simulink model "iq"  (R2021a)
settings: Solver=VariableStepAuto  StartTime=0.0  StopTime=0.2  FixedStep=1/150000  MaxStep=1e-6
undefined symbols (not defined in the file): in, ou
libraries: neural x55, spsMosfetLib x12, simulink x5, pid_lib x3, spsFirstOrderFilterLib x2, spsPermanentMagnetSynchronousMachineLib x2, spsCurrentMeasurementLib x2, spsDCVoltageSourceLib x2, spsThreePhaseVIMeasurementLib x2, spsabctoAlphaBetaZeroLib x2, spsabctodq0Lib x2, spsSVPWMGenerator2LevelLib x1
(part 1 of 5)
settings Model: Creator=Hassan Alam  LastModifiedBy=Omkar
settings SolverCC: ZeroCrossAlgorithm=Adaptive
settings DebuggingCC: MaskedZcDiagnostic=none  IgnoredZcDiagnostic=none  SFMachineParentedDataDiag=warning  ArithmeticOperatorsInVariantConditions=warning
settings SFSimCC: CustomCodeUndefinedFunction=UseInterfaceOnly

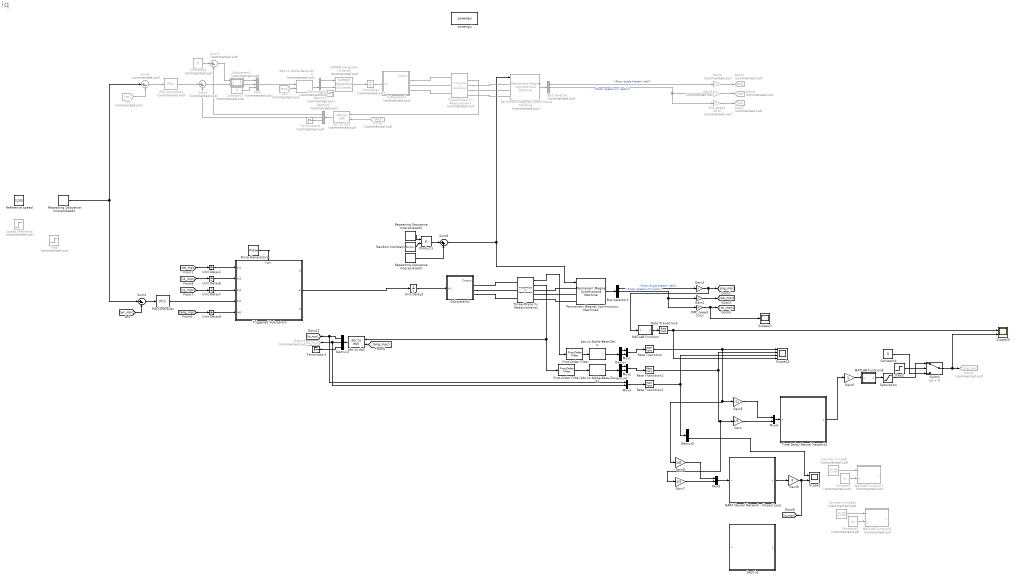
== system iq ==
  Bus Selector : BusSelector  Commented=on  OutputSignals=Rotor angle thetam (rad),Rotor speed wm (rad/s),Electromagnetic torque Te (N*m)
  Bus Selector1 : BusSelector  OutputSignals=Rotor angle thetam (rad),Rotor speed wm (rad/s),Electromagnetic torque Te (N*m)
  Constant : Constant  Commented=on  Value=in
  Constant1 : Constant  Commented=on  Value=0
  Constant2 : Constant  Commented=on  Value=0
  Constant3 : Constant  Commented=on  Value=ou
  Constant4 : Constant  Value=0
  Counter Limited : simulink/Sources/Counter Limited  Commented=on  uplimit=20000  tsamp=100e-6
  Counter Limited1 : simulink/Sources/Counter Limited  Commented=on  uplimit=20000  tsamp=10e-6
  Demux : Demux  Outputs=3
  Demux1 : Demux  Commented=on  Outputs=3
  Demux2 : Demux  Commented=on  Outputs=3
  Demux3 : Demux  Outputs=3
  Demux4 : Demux  Outputs=3
  Demux5 : Demux  Outputs=2
  FOC speed : Gain  Commented=on  Gain=30/pi
  First-Order Filter : spsFirstOrderFilterLib/First-Order Filter  FilterType=Lowpass  Tc=10e-5  Ts=0  Initialize=off  Vac_Init=[0, 0, 60]  Vdc_Init=0  PlotResponse=off  FreqRange="[0,  200,  1]"
  First-Order Filter1 : spsFirstOrderFilterLib/First-Order Filter  FilterType=Lowpass  Tc=10e-5  Ts=0  Initialize=off  Vac_Init=[0, 0, 60]  Vdc_Init=0  PlotResponse=off  FreqRange="[0,  200,  1]"
  From2 : From  Commented=on  GotoTag=ang
  Gain : Gain  Gain=1/3
  Gain1 : Gain  Commented=on  Gain=4
  Gain2 : Gain  Gain=4
  Gain3 : Gain  Gain=4
  Gain4 : Gain  Commented=on  Gain=4
  Gain5 : Gain  Gain=1/12
  Gain6 : Gain
  Gain7 : Gain  Gain=1/3
  Gain8 : Gain  Gain=1/8
  Gain9 : Gain  Gain=3
  Goto13 : Goto  Commented=on  GotoTag=iq_mpc
  Goto2 : Goto  Commented=on  GotoTag=ang
  Goto4 : Goto  Commented=on  GotoTag=we
  Goto6 : Goto  Commented=on  GotoTag=ang_mpc
  Goto7 : Goto  Commented=on  GotoTag=wr
  MATLAB Function : MATLAB Function  TreatAsAtomicUnit=on
  MATLAB Function1 : MATLAB Function  Commented=on  TreatAsAtomicUnit=on
  MATLAB Function2 : MATLAB Function  Commented=on  TreatAsAtomicUnit=on
  MATLAB Function5 : MATLAB Function  TreatAsAtomicUnit=on
  MPC speed : Gain  Gain=30/pi
  Mux : Mux  Commented=on  Inputs=3
  Mux{1..5} (5 alike) : Mux  Inputs=2
  NARX Neural Network - Closed Loop : Subsystem  mask{pi_input_1_delayed_1=[0;0;0;0], pi_input_1_delayed_2=[0;0;0;0], pi_input_1_delayed_3=[0;0;0;0], pi_input_1_delayed_4=[0;0;0;0], pi_input_1_delayed_5=[0;0;0;0], pi_input_1_delayed_6=[0;0;0;0], pi_input_1_delayed_7=[0;0;0;0], pi_input_1_delayed_8=[0;0;0;0], pi_input_1_delayed_9=[0;0;0;0], pi_input_1_delayed_10=[0;0;0;0], ai_layer_2_delayed_1=0, ai_layer_2_delayed_2=0, ai_layer_2_delayed_3=0, ai_layer_2_delayed_4=0, ai_layer_2_delayed_5=0, ai_layer_2_delayed_6=0, ai_layer_2_delayed_7=0, ai_layer_2_delayed_8=0, ai_layer_2_delayed_9=0, ai_layer_2_delayed_10=0}
      mask prompts: pi_input_1_delayed_1 "Preprocessed initial input 1 state at timestep 0."; pi_input_1_delayed_2 "Preprocessed initial input 1 state at timestep -1."; pi_input_1_delayed_3 "Preprocessed initial input 1 state at timestep -2."; pi_input_1_delayed_4 "Preprocessed initial input 1 state at timestep -3."; pi_input_1_delayed_5 "Preprocessed initial input 1 state at timestep -4."; pi_input_1_delayed_6 "Preprocessed initial input 1 state at timestep -5."; pi_input_1_delayed_7 "Preprocessed initial input 1 state at timestep -6."; pi_input_1_delayed_8 "Preprocessed initial input 1 state at timestep -7."; pi_input_1_delayed_9 "Preprocessed initial input 1 state at timestep -8."; pi_input_1_delayed_10 "Preprocessed initial input 1 state at timestep -9."; ai_layer_2_delayed_1 "Initial layer 2 state at timestep 0."; ai_layer_2_delayed_2 "Initial layer 2 state at timestep -1."; ai_layer_2_delayed_3 "Initial layer 2 state at timestep -2."; ai_layer_2_delayed_4 "Initial layer 2 state at timestep -3."; ai_layer_2_delayed_5 "Initial layer 2 state at timestep -4."; ai_layer_2_delayed_6 "Initial layer 2 state at timestep -5."; ai_layer_2_delayed_7 "Initial layer 2 state at timestep -6."; ai_layer_2_delayed_8 "Initial layer 2 state at timestep -7."; ai_layer_2_delayed_9 "Initial layer 2 state at timestep -8."; ai_layer_2_delayed_10 "Initial layer 2 state at timestep -9."
      mask help: NARX Neural Network - Closed Loop
      mask Display: e = 0.06;c1 = [120 150 230]/255;c2 = ([120 150 230]+0)/383;c3 = ([120 150 230]+128)/383;patch([0 1 1 0],[0 0 1 1],c1);patch([0 1 1 1-e 1-e 0+e],[0 0 1 1-e 0+e 0+e],c2);patch([0 0 1 1-e 0+e 0+e],[0 1 1 1-e 1-e 0+e],c3);plot([0 1 1 0 0],[0 0 1 1 0]);fprintf('NNET');port_label('input',1,' x');port_label('output',1,'y ');
  PID Controller : pid_lib/PID Controller  Controller=PI  Form=Parallel  TimeDomain=Discrete-time  UseExternalTs=off  SampleTime=1/2000  IntegratorMethod=Forward Euler  FilterMethod=Forward Euler  ControllerParametersSource=internal  P=0.02  I=20  D=0  UseFilter=on  N=100  TunerSelectOption=Transfer Function Based (PID Tuner App)  InitialConditionSource=internal  InitialConditionForIntegrator=0  InitialConditionForFilter=0  DifferentiatorICPrevScaledInput=0  ExternalReset=none  TrackingMode=off  Kt=1  LimitOutput=on  SatLimitsSource=internal  UpperSaturationLimit=3  LowerSaturationLimit=-3  LinearizeAsGain=on  AntiWindupMode=clamping  Kb=1  POutMin=[]  POutMax=[]  IOutMin=[]  IOutMax=[]  DOutMin=[]  DOutMax=[]  NOutMin=[]  NOutMax=[]  SumOutMin=[]  SumOutMax=[]  SaturationOutMin=[]  SaturationOutMax=[]  PParamMin=[]  PParamMax=[]  IParamMin=[]  IParamMax=[]  DParamMin=[]  DParamMax=[]  NParamMin=[]  NParamMax=[]  KbParamMin=[]  KbParamMax=[]  KtParamMin=[]  KtParamMax=[]  KbOutMin=[]  KbOutMax=[]  KtOutMin=[]  KtOutMax=[]  IntegratorOutMin=[]  IntegratorOutMax=[]  FilterOutMin=[]  FilterOutMax=[]  SumI1OutMin=[]  SumI1OutMax=[]  SumI2OutMin=[]  SumI2OutMax=[]  SumI3OutMin=[]  SumI3OutMax=[]  SumI4OutMin=[]  SumI4OutMax=[]  SumDOutMin=[]  SumDOutMax=[]  DifferentiatorOutMin=[]  DifferentiatorOutMax=[]  FilterDiffOutCoefMin=[]  FilterDiffOutCoefMax=[]  ReciprocalOutMin=[]  ReciprocalOutMax=[]  SumDenOutMin=[]  SumDenOutMax=[]  SumNumOutMin=[]  SumNumOutMax=[]  DivideOutMin=[]  DivideOutMax=[]  UdiffTsProdOutMin=[]  UdiffTsProdOutMax=[]  NTsProdOutMin=[]  NTsProdOutMax=[]  UintegralTsProdOutMin=[]  UintegralTsProdOutMax=[]  UngainTsProdOutMin=[]  UngainTsProdOutMax=[]  IntegratorContinuousStateAttributes=''  IntegratorStateMustResolveToSignalObject=off  IntegratorRTWStateStorageClass=Auto  FilterContinuousStateAttributes=''  FilterStateMustResolveToSignalObject=off  FilterRTWStateStorageClass=Auto  ParallelPVariant=InternalParameters  IdealPVariant=Disabled  IVariant=InternalParameters  DVariant=Disabled  IntegratorVariant=Discrete  SatVariant=Enabled  AWVariant=DiscClampingParallel  PCopyVariant=Disabled  TRVariant=Disabled  FdbkBlocksVariant=Forward  IdealPFdbkVariant=Disabled  SatFdbkVariant=Disabled  DerivativeFilterVariant=Disabled  NVariant=Disabled  NCopyVariant=Disabled_SignalSpec  FilterICVariant=Disabled  IntegratorICVariant=InternalICs  ExternalResetVariant=Disabled  TRSumVariant=Passthrough  SumFdbkVariant=Disabled  SumVariant=Sum_PI  TsampFilterVariant=InternalTs  TsampNgainVariant=Passthrough  TsampIntegralVariant=Passthrough  ExternalSaturationOutDataTypeStr=Inherit: Same as second input
  PID Controller1 : pid_lib/PID Controller  Commented=on  Controller=PI  Form=Parallel  TimeDomain=Discrete-time  UseExternalTs=off  SampleTime=1/2000  IntegratorMethod=Forward Euler  FilterMethod=Forward Euler  ControllerParametersSource=internal  P=0.02  I=20  D=0  UseFilter=on  N=100  TunerSelectOption=Transfer Function Based (PID Tuner App)  InitialConditionSource=internal  InitialConditionForIntegrator=0  InitialConditionForFilter=0  DifferentiatorICPrevScaledInput=0  ExternalReset=none  TrackingMode=off  Kt=1  LimitOutput=on  SatLimitsSource=internal  UpperSaturationLimit=3  LowerSaturationLimit=-3  LinearizeAsGain=on  AntiWindupMode=clamping  Kb=1  POutMin=[]  POutMax=[]  IOutMin=[]  IOutMax=[]  DOutMin=[]  DOutMax=[]  NOutMin=[]  NOutMax=[]  SumOutMin=[]  SumOutMax=[]  SaturationOutMin=[]  SaturationOutMax=[]  PParamMin=[]  PParamMax=[]  IParamMin=[]  IParamMax=[]  DParamMin=[]  DParamMax=[]  NParamMin=[]  NParamMax=[]  KbParamMin=[]  KbParamMax=[]  KtParamMin=[]  KtParamMax=[]  KbOutMin=[]  KbOutMax=[]  KtOutMin=[]  KtOutMax=[]  IntegratorOutMin=[]  IntegratorOutMax=[]  FilterOutMin=[]  FilterOutMax=[]  SumI1OutMin=[]  SumI1OutMax=[]  SumI2OutMin=[]  SumI2OutMax=[]  SumI3OutMin=[]  SumI3OutMax=[]  SumI4OutMin=[]  SumI4OutMax=[]  SumDOutMin=[]  SumDOutMax=[]  DifferentiatorOutMin=[]  DifferentiatorOutMax=[]  FilterDiffOutCoefMin=[]  FilterDiffOutCoefMax=[]  ReciprocalOutMin=[]  ReciprocalOutMax=[]  SumDenOutMin=[]  SumDenOutMax=[]  SumNumOutMin=[]  SumNumOutMax=[]  DivideOutMin=[]  DivideOutMax=[]  UdiffTsProdOutMin=[]  UdiffTsProdOutMax=[]  NTsProdOutMin=[]  NTsProdOutMax=[]  UintegralTsProdOutMin=[]  UintegralTsProdOutMax=[]  UngainTsProdOutMin=[]  UngainTsProdOutMax=[]  IntegratorContinuousStateAttributes=''  IntegratorStateMustResolveToSignalObject=off  IntegratorRTWStateStorageClass=Auto  FilterContinuousStateAttributes=''  FilterStateMustResolveToSignalObject=off  FilterRTWStateStorageClass=Auto  ParallelPVariant=InternalParameters  IdealPVariant=Disabled  IVariant=InternalParameters  DVariant=Disabled  IntegratorVariant=Discrete  SatVariant=Enabled  AWVariant=DiscClampingParallel  PCopyVariant=Disabled  TRVariant=Disabled  FdbkBlocksVariant=Forward  IdealPFdbkVariant=Disabled  SatFdbkVariant=Disabled  DerivativeFilterVariant=Disabled  NVariant=Disabled  NCopyVariant=Disabled_SignalSpec  FilterICVariant=Disabled  IntegratorICVariant=InternalICs  ExternalResetVariant=Disabled  TRSumVariant=Passthrough  SumFdbkVariant=Disabled  SumVariant=Sum_PI  TsampFilterVariant=InternalTs  TsampNgainVariant=Passthrough  TsampIntegralVariant=Passthrough  ExternalSaturationOutDataTypeStr=Inherit: Same as second input
  Permanent Magnet Synchronous Machine : spsPermanentMagnetSynchronousMachineLib/Permanent Magnet Synchronous Machine  Commented=on  NbPhases=3  FluxDistribution=Sinusoidal  RotorType=Round  MechanicalLoad=Torque Tm  PresetModel=No  ShowDetailedParameters=on  MeasurementBus=off  Resistance=0.75  Inductance=8.5e-3  dqInductances=[8.5e-3,8.5e-3]  La=0.0004  MachineConstant=Flux linkage established by magnets (V.s)  Flux=0.00666  VoltageCst=4.832  TorqueCst=0.03996  Flat=120  Mechanical=[2.66e-6 1.33e-6 4 0]  PolePairs=4  InitialConditions=[0,0, 0,0]  InitialConditions5ph=[0 0 0 0 0 0]  RefAngle=90 degrees behind phase A axis (modified Park)  IterativeDiscreteModel=Trapezoidal non iterative  TsBlock=-1  TsPowergui=0
  Permanent Magnet Synchronous Machine2 : spsPermanentMagnetSynchronousMachineLib/Permanent Magnet Synchronous Machine  NbPhases=3  FluxDistribution=Sinusoidal  RotorType=Round  MechanicalLoad=Torque Tm  PresetModel=No  ShowDetailedParameters=on  MeasurementBus=off  Resistance=0.75  Inductance=8.5e-3  dqInductances=[8.5e-3,8.5e-3]  La=0.0004  MachineConstant=Flux linkage established by magnets (V.s)  Flux=0.00666  VoltageCst=4.832  TorqueCst=0.03996  Flat=120  Mechanical=[2.66e-6 1.33e-6 4 0]  PolePairs=4  InitialConditions=[0,0, 0,0]  InitialConditions5ph=[0 0 0 0 0 0]  RefAngle=90 degrees behind phase A axis (modified Park)  IterativeDiscreteModel=Trapezoidal non iterative  TsBlock=-1  TsPowergui=0
  Product1 : Product
  Pulse Generator1 : DiscretePulseGenerator  PulseType=Time based  Period=1/40000  PulseWidth=5
  Qr1 : From  Commented=on  GotoTag=wr
  Qr2 : From  Commented=on  GotoTag=ang
  Random Number1 : RandomNumber  Mean=0.5  Seed=123  SampleTime=1e-5
  Rate Transition{,1..3} (4 alike) : RateTransition  OutPortSampleTime=10e-6
  Reference speed : Constant  Value=1200
  Repeating Sequence Interpolated2 : simulink/Sources/Repeating Sequence Interpolated  OutValues=[1500 1500 1000 1000 1200 1200 1000 1000 1000 1000 1500 1500 0].'  TimeValues=[0 0.0229 0.023 0.0499 0.05 0.095 0.10 0.159 0.16 0.20 0.22 0.27 0.3].'/3  LookUpMeth=Interpolation-Use End Values  tsamp=1e-6  OutMin=[]  OutMax=[]  OutDataTypeStr=double  OutputDataTypeScalingMode=double  OutDataType=fixdt(0,8)  OutScaling=2^-10
  Repeating Sequence Interpolated3 : simulink/Sources/Repeating Sequence Interpolated  OutValues=[0 0.05 0.05 0.1 0.1 0.125 0.125 0.05 0].'*0.9  TimeValues=[0 0.01 0.02 0.05 0.15 0.16 0.25 0.27 0.3].'/6  LookUpMeth=Interpolation-Use End Values  tsamp=1e-6  OutMin=[]  OutMax=[]  OutDataTypeStr=double  OutputDataTypeScalingMode=double  OutDataType=fixdt(0,8)  OutScaling=2^-10
  Repeating Sequence Interpolated4 : simulink/Sources/Repeating Sequence Interpolated  OutValues=[0 0.008 0.008 0.015 0.015 0.02 0.02 0.008 0].'  TimeValues=[0 0.01 0.02 0.05 0.15 0.16 0.25 0.27 0.3].'/6  LookUpMeth=Interpolation-Use End Values  tsamp=1e-6  OutMin=[]  OutMax=[]  OutDataTypeStr=double  OutputDataTypeScalingMode=double  OutDataType=fixdt(0,8)  OutScaling=2^-10
  SVPWM Generator (2-Level) : spsSVPWMGenerator2LevelLib/SVPWM Generator (2-Level)  Commented=on  InputType=alpha-beta components  SwitchingPattern=Pattern #1  Fc=40000  ParUref=[0.8 -30 50]  Ts=0
      settings: SourceProductBaseCode=PS
  Saturation : Saturate  UpperLimit=2*pi  LowerLimit=0
  Scope1 : Scope  NumInputPorts=2
  Scope14 : Scope  NumInputPorts=4
  Scope20 : Scope  NumInputPorts=2
  Scope21 : Scope
  Speed reference : Step  Commented=on  Time=0.2  Before=1500  After=-1500  SampleTime=0
  Step : Step  Commented=on  Time=0  After=800  SampleTime=0
  Step2 : Step  Time=2e-3  SampleTime=0
  Subsystem1 : Subsystem  Commented=on
  Subsystem2 : Subsystem
  Subsystem3 : Subsystem  Commented=on
  Sum1 : Sum  Commented=on  Inputs=|+-
  Sum2 : Sum  Inputs=|+-
  Sum3 : Sum  Commented=on  Inputs=|+-
  Sum5 : Sum  Commented=on  Inputs=|+-
  Sum9 : Sum  Inputs=|++
  Switch : Switch  Criteria=u2 > Threshold
  Terminator1 : Terminator
  Terminator2 : Terminator  Commented=on
  Terminator3 : Terminator  Commented=on
  Three-Phase V-I Measurement : spsThreePhaseVIMeasurementLib/Three-Phase V-I Measurement  Commented=on  VoltageMeasurement=phase-to-phase  SetLabelV=off  LabelV=Vabc  Vpu=off  VpuLL=off  CurrentMeasurement=yes  SetLabelI=off  LabelI=Iabc  Ipu=off  Pbase=100e6  Vbase=500e3  OutputType=Complex  PhasorSimulation=off  PSBequivalent=0
  Three-Phase V-I Measurement1 : spsThreePhaseVIMeasurementLib/Three-Phase V-I Measurement  VoltageMeasurement=phase-to-phase  SetLabelV=off  LabelV=Vabc  Vpu=off  VpuLL=off  CurrentMeasurement=yes  SetLabelI=off  LabelI=Iabc  Ipu=off  Pbase=100e6  Vbase=500e3  OutputType=Complex  PhasorSimulation=off  PSBequivalent=0
  Time Delay Neural Network1 : Subsystem  mask{pi_input_1_delayed_1=[0;0;0;0], pi_input_1_delayed_2=[0;0;0;0], pi_input_1_delayed_3=[0;0;0;0], pi_input_1_delayed_4=[0;0;0;0], pi_input_1_delayed_5=[0;0;0;0], pi_input_1_delayed_6=[0;0;0;0], pi_input_1_delayed_7=[0;0;0;0], pi_input_1_delayed_8=[0;0;0;0], pi_input_1_delayed_9=[0;0;0;0], pi_input_1_delayed_10=[0;0;0;0]}
      mask prompts: pi_input_1_delayed_1 "Preprocessed initial input 1 state at timestep 0."; pi_input_1_delayed_2 "Preprocessed initial input 1 state at timestep -1."; pi_input_1_delayed_3 "Preprocessed initial input 1 state at timestep -2."; pi_input_1_delayed_4 "Preprocessed initial input 1 state at timestep -3."; pi_input_1_delayed_5 "Preprocessed initial input 1 state at timestep -4."; pi_input_1_delayed_6 "Preprocessed initial input 1 state at timestep -5."; pi_input_1_delayed_7 "Preprocessed initial input 1 state at timestep -6."; pi_input_1_delayed_8 "Preprocessed initial input 1 state at timestep -7."; pi_input_1_delayed_9 "Preprocessed initial input 1 state at timestep -8."; pi_input_1_delayed_10 "Preprocessed initial input 1 state at timestep -9."
      mask help: Time Delay Neural Network
      mask Display: e = 0.06;c1 = [120 150 230]/255;c2 = ([120 150 230]+0)/383;c3 = ([120 150 230]+128)/383;patch([0 1 1 0],[0 0 1 1],c1);patch([0 1 1 1-e 1-e 0+e],[0 0 1 1-e 0+e 0+e],c2);patch([0 0 1 1-e 0+e 0+e],[0 1 1 1-e 1-e 0+e],c3);plot([0 1 1 0 0],[0 0 1 1 0]);fprintf('NNET');port_label('input',1,' x');port_label('output',1,'y ');
  Triggered Subsystem : Subsystem  TreatAsAtomicUnit=on
  Unit Delay : UnitDelay  Commented=on  SampleTime=1e-6  HasFrameUpgradeWarning=on
  Unit Delay{1,6..7,9} (4 alike) : UnitDelay  SampleTime=-1  HasFrameUpgradeWarning=on
  Unit Delay2 : UnitDelay  SampleTime=1e-6  HasFrameUpgradeWarning=on
  abc to Alpha-Beta-Zero : spsabctoAlphaBetaZeroLib/abc to Alpha-Beta-Zero
      settings: SourceProductBaseCode=PS
  abc to Alpha-Beta-Zero1 : spsabctoAlphaBetaZeroLib/abc to Alpha-Beta-Zero
      settings: SourceProductBaseCode=PS
  abc to dq1 : spsabctodq0Lib/abc to dq0  Alignment=90 degrees behind phase A axis
  abc to dq2 : spsabctodq0Lib/abc to dq0  Commented=on  Alignment=90 degrees behind phase A axis
  best iq : Subsystem  mask{pi_input_1_delayed_1=[0;0;0;0], pi_input_1_delayed_2=[0;0;0;0], pi_input_1_delayed_3=[0;0;0;0], pi_input_1_delayed_4=[0;0;0;0], pi_input_1_delayed_5=[0;0;0;0], ai_layer_2_delayed_1=0, ai_layer_2_delayed_2=0, ai_layer_2_delayed_3=0, ai_layer_2_delayed_4=0, ai_layer_2_delayed_5=0}
      mask prompts: pi_input_1_delayed_1 "Preprocessed initial input 1 state at timestep 0."; pi_input_1_delayed_2 "Preprocessed initial input 1 state at timestep -1."; pi_input_1_delayed_3 "Preprocessed initial input 1 state at timestep -2."; pi_input_1_delayed_4 "Preprocessed initial input 1 state at timestep -3."; pi_input_1_delayed_5 "Preprocessed initial input 1 state at timestep -4."; ai_layer_2_delayed_1 "Initial layer 2 state at timestep 0."; ai_layer_2_delayed_2 "Initial layer 2 state at timestep -1."; ai_layer_2_delayed_3 "Initial layer 2 state at timestep -2."; ai_layer_2_delayed_4 "Initial layer 2 state at timestep -3."; ai_layer_2_delayed_5 "Initial layer 2 state at timestep -4."
      mask help: NARX Neural Network - Closed Loop
      mask Display: e = 0.06;c1 = [120 150 230]/255;c2 = ([120 150 230]+0)/383;c3 = ([120 150 230]+128)/383;patch([0 1 1 0],[0 0 1 1],c1);patch([0 1 1 1-e 1-e 0+e],[0 0 1 1-e 0+e 0+e],c2);patch([0 0 1 1-e 0+e 0+e],[0 1 1 1-e 1-e 0+e],c3);plot([0 1 1 0 0],[0 0 1 1 0]);fprintf('NNET');port_label('input',1,' x');port_label('output',1,'y ');
  dq0 to Alpha-Beta-Zero : spsdq0toAlphaBetaZeroLib/dq0 to Alpha-Beta-Zero  Commented=on  Alignment=90 degrees behind phase A axis
      settings: SourceProductBaseCode=PS
  powergui : spspowerguiLib/powergui  Priority=1  SimulationMode=Discrete  SampleTime=10e-6  frequency=60  Iterations=50  frequencyindice=0  Pbase=100e6  ErrMax=1e-4  UnitsV=kV  UnitsW=MW  buscounter=0  FunctionMessages=off  echomessages=off  EnableUseOfTLC=off  CurrentSourceSwitches=off  DisableSnubberDevices=off  DisableRonSwitches=off  DisableVfSwitches=off  DisplayEquations=off  AutomaticDiscreteSolvers=off  SolverType=Tustin/Backward Euler (TBE)  Interpol=off  ExternalGateDelay=off  methode=off  Ts=100  x0status=blocks  SPID=on  SwTol=0  HookPort=off  NonlinearTolerance=1e-4  nMaxIteration=100  ContinueOnMaxIteration=off  RestoreLinks=warning  ResistiveCurrentMeasurement=off  Frange=[0:2:500]  Ylog=off  Xlog=on  ShowGrid=off  save=off  variable=ZData  structure=0  ZoomFFT=off  StartTime=0.0  cycles=1  DisplayStyle=1  fundamental=60  FreqAxis=off  MaxFrequency=1000  frequencyindicesteady=1  RmsSteady=1  display=off
  wires:
  Qr1/1 -> Sum5/2
  Unit Delay7/1 -> Triggered Subsystem/3(In4)
  [we_mpc] -> Unit Delay1/1
  [ang_mpc] -> Unit Delay9/1
  [iq_mpc] -> Unit Delay7/1
  PID Controller/1 -> Triggered Subsystem/4(In5)
  Unit Delay1/1 -> Triggered Subsystem/1(In1)
  [id_mpc] -> Unit Delay6/1
  Unit Delay6/1 -> Triggered Subsystem/2(In3)
  Unit Delay9/1 -> Triggered Subsystem/5(In6)
  Pulse Generator1/1 -> Triggered Subsystem/Trigger
  Constant2/1 -> Sum1/1
  dq0 to Alpha-Beta-Zero/1 -> Demux1/1
  Demux1/2 -> SVPWM Generator (2-Level)/2
  Demux1/1 -> SVPWM Generator (2-Level)/1
  Demux1/3 -> Terminator2/1
  Qr2/1 -> dq0 to Alpha-Beta-Zero/2
  Constant1/1 -> Mux/3
  abc to dq2/1 -> Demux2/1
  Gain4/1 -> Goto2/1
  Gain1/1 -> Goto4/1
  From2/1 -> abc to dq2/2
  Demux2/3 -> Terminator3/1
  Demux3/3 -> Terminator1/1
  [ang_mpc] -> abc to dq1/2
  abc to dq1/1 -> Demux3/1
  Three-Phase V-I Measurement1/2 -> First-Order Filter1/1, abc to dq1/1
  Three-Phase V-I Measurement/2 -> abc to dq2/1
  Demux2/2 -> Sum3/2
  Demux3/2 -> Mux3/2, Goto13/1
  Demux3/1 -> Mux3/1, [id_mpc]
  Demux2/1 -> Sum1/2
  Three-Phase V-I Measurement1/1 -> First-Order Filter/1
  Sum5/1 -> PID Controller1/1
  Repeating Sequence Interpolated2/1 -> Sum5/1, Sum2/1
  [wr_mpc] -> Sum2/2
  Sum1/1 -> Subsystem1/1(In1)
  Sum3/1 -> Subsystem1/2(In2)
  Subsystem1/1(Out1) -> Mux/1
  Subsystem1/2(Out2) -> Mux/2
  Sum2/1 -> PID Controller/1
  Sum9/1 -> Permanent Magnet Synchronous Machine2/1, Permanent Magnet Synchronous Machine/1
  PID Controller1/1 -> Sum3/1
  Mux/1 -> dq0 to Alpha-Beta-Zero/1
  SVPWM Generator (2-Level)/1 -> Unit Delay/1
  Unit Delay/1 -> Subsystem3/1(In1)
  Permanent Magnet Synchronous Machine/1 -> Bus Selector/1
  Bus Selector/1 -> Gain4/1  "<Rotor angle thetam (rad)>"
  Bus Selector/2 -> FOC speed/1, Gain1/1  "<Rotor speed wm (rad/s)>"
  Bus Selector1/2 -> Gain2/1, MPC speed/1  "<Rotor speed wm (rad/s)>"
  Bus Selector1/1 -> Gain3/1  "<Rotor angle thetam (rad)>"
  Permanent Magnet Synchronous Machine2/1 -> Bus Selector1/1
  Gain2/1 -> [we_mpc]
  Gain3/1 -> MATLAB Function/1(u), [ang_mpc]
  Unit Delay2/1 -> Subsystem2/1(In1)
  FOC speed/1 -> Goto7/1
  MPC speed/1 -> Scope21/1, [wr_mpc]
  Random Number1/1 -> Product1/2
  Repeating Sequence Interpolated4/1 -> Product1/1
  Repeating Sequence Interpolated3/1 -> Sum9/2
  Product1/1 -> Sum9/1
  Triggered Subsystem/2(a) -> Unit Delay2/1
  Demux4/1 -> Mux2/1
  Demux4/2 -> Mux2/2
  abc to Alpha-Beta-Zero/1 -> Demux/1
  Demux/1 -> Mux1/1
  abc to Alpha-Beta-Zero1/1 -> Demux4/1
  Demux/2 -> Mux1/2
  Mux1/1 -> Rate Transition/1
  Mux2/1 -> Rate Transition1/1
  Mux3/1 -> Rate Transition2/1
  MATLAB Function/1(y) -> Rate Transition3/1
  First-Order Filter/1 -> abc to Alpha-Beta-Zero/1
  First-Order Filter1/1 -> abc to Alpha-Beta-Zero1/1
  Rate Transition/1 -> Gain8/1, Gain5/1, Scope14/1
  Rate Transition2/1 -> Scope14/3, Demux5/1
  Rate Transition1/1 -> Scope14/2, Gain7/1, Gain/1
  Rate Transition3/1 -> Scope14/4, Scope20/1
  Constant/1 -> MATLAB Function1/2(u)
  Counter Limited/1 -> MATLAB Function1/1(i)
  Counter Limited1/1 -> MATLAB Function2/1(i)
  Constant3/1 -> MATLAB Function2/2(u)
  Mux4/1 -> Time Delay Neural Network1/1(x)
  Gain/1 -> Mux4/2
  Gain5/1 -> Mux4/1
  Time Delay Neural Network1/1(y) -> Gain6/1
  Switch/1 -> Scope20/2, Goto6/1
  Step2/1 -> Switch/2
  Saturation/1 -> Switch/1
  Constant4/1 -> Switch/3
  Gain6/1 -> MATLAB Function5/1(u)
  MATLAB Function5/1(y) -> Saturation/1
  Gain8/1 -> Mux5/1
  Gain7/1 -> Mux5/2
  NARX Neural Network - Closed Loop/1(y) -> Gain9/1
  Demux5/2 -> Scope1/1
  Gain9/1 -> Scope1/2, [iq_mpc]
  Mux5/1 -> NARX Neural Network - Closed Loop/1(x)
  connections:
  Subsystem3/RConn1 -- Three-Phase V-I Measurement/LConn1
  Subsystem3/RConn2 -- Three-Phase V-I Measurement/LConn2
  Subsystem3/RConn3 -- Three-Phase V-I Measurement/LConn3
  Three-Phase V-I Measurement/RConn1 -- Permanent Magnet Synchronous Machine/LConn1
  Three-Phase V-I Measurement/RConn2 -- Permanent Magnet Synchronous Machine/LConn2
  Three-Phase V-I Measurement/RConn3 -- Permanent Magnet Synchronous Machine/LConn3
  Permanent Magnet Synchronous Machine2/LConn3 -- Three-Phase V-I Measurement1/RConn3
  Permanent Magnet Synchronous Machine2/LConn1 -- Three-Phase V-I Measurement1/RConn1
  Subsystem2/RConn2 -- Three-Phase V-I Measurement1/LConn2
  Subsystem2/RConn3 -- Three-Phase V-I Measurement1/LConn3
  Three-Phase V-I Measurement1/LConn1 -- Subsystem2/RConn1
  Permanent Magnet Synchronous Machine2/LConn2 -- Three-Phase V-I Measurement1/RConn2

== system iq/NARX Neural Network - Closed Loop ==
  x : Inport  PortDimensions=4  SampleTime=1e-05
      mask Display: e = 0.06;c1 = [120 230 180]/255;c2 = ([120 230 180]+0)/(256+128);c3 = ([120 230 180]+128)/(256+128);patch([0 1 1 0],[0 0 1 1],c1);patch([0 1 1 1-e 1-e 0+e],[0 0 1 1-e 0+e 0+e],c2);patch([0 0 1 1-e 0+e 0+e],[0 1 1 1-e 1-e 0+e],c3);plot([0 1 1 0 0],[0 0 1 1 0]);
  Layer 1 : Subsystem
      mask Display: e = 0.06;c1 = [120 150 230]/255;c2 = ([120 150 230]+0)/383;c3 = ([120 150 230]+128)/383;patch([0 1 1 0],[0 0 1 1],c1);patch([0 1 1 1-e 1-e 0+e],[0 0 1 1-e 0+e 0+e],c2);patch([0 0 1 1-e 0+e 0+e],[0 1 1 1-e 1-e 0+e],c3);plot([0 1 1 0 0],[0 0 1 1 0]);
  Layer 2 : Subsystem
      mask Display: e = 0.06;c1 = [120 150 230]/255;c2 = ([120 150 230]+0)/383;c3 = ([120 150 230]+128)/383;patch([0 1 1 0],[0 0 1 1],c1);patch([0 1 1 1-e 1-e 0+e],[0 0 1 1-e 0+e 0+e],c2);patch([0 0 1 1-e 0+e 0+e],[0 1 1 1-e 1-e 0+e],c3);plot([0 1 1 0 0],[0 0 1 1 0]);
  Process Input 1 : Subsystem
      mask Display: e = 0.06;c1 = [120 150 230]/255;c2 = ([120 150 230]+0)/383;c3 = ([120 150 230]+128)/383;patch([0 1 1 0],[0 0 1 1],c1);patch([0 1 1 1-e 1-e 0+e],[0 0 1 1-e 0+e 0+e],c2);patch([0 0 1 1-e 0+e 0+e],[0 1 1 1-e 1-e 0+e],c3);plot([0 1 1 0 0],[0 0 1 1 0]);
  Process Output 1 : Subsystem
      mask Display: e = 0.06;c1 = [120 150 230]/255;c2 = ([120 150 230]+0)/383;c3 = ([120 150 230]+128)/383;patch([0 1 1 0],[0 0 1 1],c1);patch([0 1 1 1-e 1-e 0+e],[0 0 1 1-e 0+e 0+e],c2);patch([0 0 1 1-e 0+e 0+e],[0 1 1 1-e 1-e 0+e],c3);plot([0 1 1 0 0],[0 0 1 1 0]);
  y : Outport  InitialOutput=0
      mask Display: e = 0.06;c1 = [120 230 180]/255;c2 = ([120 230 180]+0)/(256+128);c3 = ([120 230 180]+128)/(256+128);patch([0 1 1 0],[0 0 1 1],c1);patch([0 1 1 1-e 1-e 0+e],[0 0 1 1-e 0+e 0+e],c2);patch([0 0 1 1-e 0+e 0+e],[0 1 1 1-e 1-e 0+e],c3);plot([0 1 1 0 0],[0 0 1 1 0]);
  wires:
  x/1 -> Process Input 1/1(x)
  Process Output 1/1(y) -> y/1
  Process Input 1/1(p) -> Layer 1/1("p{1}")
  Layer 1/1("a{1}") -> [feedback1]
  [feedback1] -> Layer 2/1("a{1} ")
  Layer 2/1("a{2}") -> [feedback2], Process Output 1/1(a)
  [feedback2] -> Layer 1/2("a{2} ")

== system iq/Subsystem1 ==
  In1 : Inport
  In2 : Inport  Port=2
  Demux : Demux  Outputs=2
  Mux1 : Mux  Inputs=2
  PID Controller1 : pid_lib/PID Controller  Controller=PI  Form=Parallel  TimeDomain=Discrete-time  UseExternalTs=off  SampleTime=1/40000  IntegratorMethod=Forward Euler  FilterMethod=Forward Euler  ControllerParametersSource=internal  P=1  I=800  D=0  UseFilter=on  N=100  TunerSelectOption=Transfer Function Based (PID Tuner App)  InitialConditionSource=internal  InitialConditionForIntegrator=0  InitialConditionForFilter=0  DifferentiatorICPrevScaledInput=0  ExternalReset=none  TrackingMode=off  Kt=1  LimitOutput=off  SatLimitsSource=internal  UpperSaturationLimit=3  LowerSaturationLimit=-3  LinearizeAsGain=on  AntiWindupMode=clamping  Kb=1  POutMin=[]  POutMax=[]  IOutMin=[]  IOutMax=[]  DOutMin=[]  DOutMax=[]  NOutMin=[]  NOutMax=[]  SumOutMin=[]  SumOutMax=[]  SaturationOutMin=[]  SaturationOutMax=[]  PParamMin=[]  PParamMax=[]  IParamMin=[]  IParamMax=[]  DParamMin=[]  DParamMax=[]  NParamMin=[]  NParamMax=[]  KbParamMin=[]  KbParamMax=[]  KtParamMin=[]  KtParamMax=[]  KbOutMin=[]  KbOutMax=[]  KtOutMin=[]  KtOutMax=[]  IntegratorOutMin=[]  IntegratorOutMax=[]  FilterOutMin=[]  FilterOutMax=[]  SumI1OutMin=[]  SumI1OutMax=[]  SumI2OutMin=[]  SumI2OutMax=[]  SumI3OutMin=[]  SumI3OutMax=[]  SumI4OutMin=[]  SumI4OutMax=[]  SumDOutMin=[]  SumDOutMax=[]  DifferentiatorOutMin=[]  DifferentiatorOutMax=[]  FilterDiffOutCoefMin=[]  FilterDiffOutCoefMax=[]  ReciprocalOutMin=[]  ReciprocalOutMax=[]  SumDenOutMin=[]  SumDenOutMax=[]  SumNumOutMin=[]  SumNumOutMax=[]  DivideOutMin=[]  DivideOutMax=[]  UdiffTsProdOutMin=[]  UdiffTsProdOutMax=[]  NTsProdOutMin=[]  NTsProdOutMax=[]  UintegralTsProdOutMin=[]  UintegralTsProdOutMax=[]  UngainTsProdOutMin=[]  UngainTsProdOutMax=[]  IntegratorContinuousStateAttributes=''  IntegratorStateMustResolveToSignalObject=off  IntegratorRTWStateStorageClass=Auto  FilterContinuousStateAttributes=''  FilterStateMustResolveToSignalObject=off  FilterRTWStateStorageClass=Auto  ParallelPVariant=InternalParameters  IdealPVariant=Disabled  IVariant=InternalParameters  DVariant=Disabled  IntegratorVariant=Discrete  SatVariant=Disabled  AWVariant=Passthrough  PCopyVariant=Disabled  TRVariant=Disabled  FdbkBlocksVariant=Forward  IdealPFdbkVariant=Disabled  SatFdbkVariant=Disabled  DerivativeFilterVariant=Disabled  NVariant=Disabled  NCopyVariant=Disabled_SignalSpec  FilterICVariant=Disabled  IntegratorICVariant=InternalICs  ExternalResetVariant=Disabled  TRSumVariant=Passthrough  SumFdbkVariant=Disabled  SumVariant=Sum_PI  TsampFilterVariant=InternalTs  TsampNgainVariant=Passthrough  TsampIntegralVariant=Passthrough  ExternalSaturationOutDataTypeStr=Inherit: Same as second input
  Out1 : Outport
  Out2 : Outport  Port=2
  wires:
  In1/1 -> Mux1/1
  Mux1/1 -> PID Controller1/1
  Demux/2 -> Out2/1
  PID Controller1/1 -> Demux/1
  Demux/1 -> Out1/1
  In2/1 -> Mux1/2

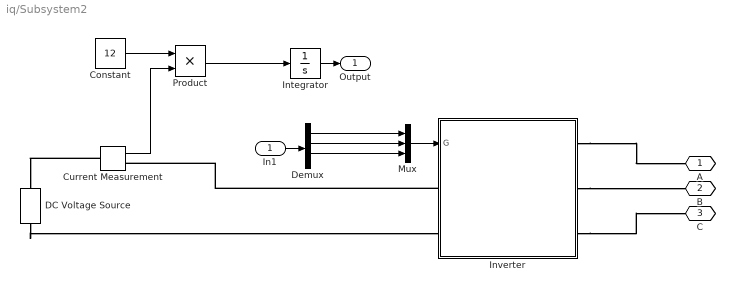
== system iq/Subsystem2 ==
  In1 : Inport
  Constant : Constant  Value=12
  Current Measurement : spsCurrentMeasurementLib/Current Measurement  PhasorSimulation=off  OutputType=Complex  PSBequivalent=0
  DC Voltage Source : spsDCVoltageSourceLib/DC Voltage Source  Amplitude=12  Measurements=None
  Demux : Demux  Outputs=6
  Integrator : Integrator
  Inverter : Subsystem
  Mux : Mux  Inputs=3
  Product : Product
  A : PMIOPort  Side=Right
  B : PMIOPort  Port=2  Side=Right
  C : PMIOPort  Port=3  Side=Right
  Output : Outport
  wires:
  Current Measurement/1 -> Product/2
  Integrator/1 -> Output/1
  Constant/1 -> Product/1
  Product/1 -> Integrator/1
  Demux/5 -> Mux/3
  Mux/1 -> Inverter/1(G)
  Demux/1 -> Mux/1
  Demux/3 -> Mux/2
  In1/1 -> Demux/1
  connections:
  Inverter/LConn1 -- Current Measurement/RConn1
  DC Voltage Source/LConn1 -- Inverter/LConn2
  Current Measurement/LConn1 -- DC Voltage Source/RConn1
  Inverter/RConn1 -- A/RConn1
  Inverter/RConn2 -- B/RConn1
  Inverter/RConn3 -- C/RConn1

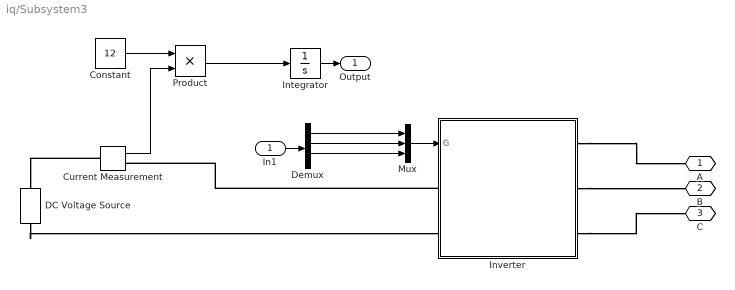
== system iq/Subsystem3 ==
  In1 : Inport
  Constant : Constant  Value=12
  Current Measurement : spsCurrentMeasurementLib/Current Measurement  PhasorSimulation=off  OutputType=Complex  PSBequivalent=0
  DC Voltage Source : spsDCVoltageSourceLib/DC Voltage Source  Amplitude=12  Measurements=None
  Demux : Demux  Outputs=6
  Integrator : Integrator
  Inverter : Subsystem
  Mux : Mux  Inputs=3
  Product : Product
  A : PMIOPort  Side=Right
  B : PMIOPort  Port=2  Side=Right
  C : PMIOPort  Port=3  Side=Right
  Output : Outport
  wires:
  In1/1 -> Demux/1
  Demux/3 -> Mux/2
  Demux/1 -> Mux/1
  Mux/1 -> Inverter/1(G)
  Demux/5 -> Mux/3
  Product/1 -> Integrator/1
  Constant/1 -> Product/1
  Integrator/1 -> Output/1
  Current Measurement/1 -> Product/2
  connections:
  Inverter/RConn3 -- C/RConn1
  Inverter/RConn2 -- B/RConn1
  Inverter/RConn1 -- A/RConn1
  Current Measurement/LConn1 -- DC Voltage Source/RConn1
  DC Voltage Source/LConn1 -- Inverter/LConn2
  Inverter/LConn1 -- Current Measurement/RConn1

== system iq/Time Delay Neural Network1 ==
  x : Inport  PortDimensions=4  SampleTime=1e-05
      mask Display: e = 0.06;c1 = [120 230 180]/255;c2 = ([120 230 180]+0)/(256+128);c3 = ([120 230 180]+128)/(256+128);patch([0 1 1 0],[0 0 1 1],c1);patch([0 1 1 1-e 1-e 0+e],[0 0 1 1-e 0+e 0+e],c2);patch([0 0 1 1-e 0+e 0+e],[0 1 1 1-e 1-e 0+e],c3);plot([0 1 1 0 0],[0 0 1 1 0]);
  Layer 1 : Subsystem
      mask Display: e = 0.06;c1 = [120 150 230]/255;c2 = ([120 150 230]+0)/383;c3 = ([120 150 230]+128)/383;patch([0 1 1 0],[0 0 1 1],c1);patch([0 1 1 1-e 1-e 0+e],[0 0 1 1-e 0+e 0+e],c2);patch([0 0 1 1-e 0+e 0+e],[0 1 1 1-e 1-e 0+e],c3);plot([0 1 1 0 0],[0 0 1 1 0]);
  Layer 2 : Subsystem
      mask Display: e = 0.06;c1 = [120 150 230]/255;c2 = ([120 150 230]+0)/383;c3 = ([120 150 230]+128)/383;patch([0 1 1 0],[0 0 1 1],c1);patch([0 1 1 1-e 1-e 0+e],[0 0 1 1-e 0+e 0+e],c2);patch([0 0 1 1-e 0+e 0+e],[0 1 1 1-e 1-e 0+e],c3);plot([0 1 1 0 0],[0 0 1 1 0]);
  Process Input 1 : Subsystem
      mask Display: e = 0.06;c1 = [120 150 230]/255;c2 = ([120 150 230]+0)/383;c3 = ([120 150 230]+128)/383;patch([0 1 1 0],[0 0 1 1],c1);patch([0 1 1 1-e 1-e 0+e],[0 0 1 1-e 0+e 0+e],c2);patch([0 0 1 1-e 0+e 0+e],[0 1 1 1-e 1-e 0+e],c3);plot([0 1 1 0 0],[0 0 1 1 0]);
  Process Output 1 : Subsystem
      mask Display: e = 0.06;c1 = [120 150 230]/255;c2 = ([120 150 230]+0)/383;c3 = ([120 150 230]+128)/383;patch([0 1 1 0],[0 0 1 1],c1);patch([0 1 1 1-e 1-e 0+e],[0 0 1 1-e 0+e 0+e],c2);patch([0 0 1 1-e 0+e 0+e],[0 1 1 1-e 1-e 0+e],c3);plot([0 1 1 0 0],[0 0 1 1 0]);
  y : Outport  InitialOutput=0
      mask Display: e = 0.06;c1 = [120 230 180]/255;c2 = ([120 230 180]+0)/(256+128);c3 = ([120 230 180]+128)/(256+128);patch([0 1 1 0],[0 0 1 1],c1);patch([0 1 1 1-e 1-e 0+e],[0 0 1 1-e 0+e 0+e],c2);patch([0 0 1 1-e 0+e 0+e],[0 1 1 1-e 1-e 0+e],c3);plot([0 1 1 0 0],[0 0 1 1 0]);
  wires:
  x/1 -> Process Input 1/1(x)
  Process Output 1/1(y) -> y/1
  Process Input 1/1(p) -> Layer 1/1("p{1}")
  Layer 1/1("a{1}") -> [feedback1]
  [feedback1] -> Layer 2/1("a{1} ")
  Layer 2/1("a{2}") -> Process Output 1/1(a)

== system iq/Triggered Subsystem ==
  In1 : Inport
  In3 : Inport  Port=2
  In4 : Inport  Port=3
  In5 : Inport  Port=4
  In6 : Inport  Port=5
  Trigger : TriggerPort  VariantControl=Variant
  MATLAB Function2 : MATLAB Function  TreatAsAtomicUnit=on
  Scope : Scope
  d : Outport  VectorParamsAs1DForOutWhenUnconnected=off
  a : Outport  Port=2  VectorParamsAs1DForOutWhenUnconnected=off
  b : Outport  Port=3  VectorParamsAs1DForOutWhenUnconnected=off
  wires:
  In1/1 -> MATLAB Function2/1(we)
  In3/1 -> MATLAB Function2/2(id)
  In4/1 -> MATLAB Function2/3(iq)
  In5/1 -> MATLAB Function2/4(iqref)
  In6/1 -> MATLAB Function2/5(ang)
  MATLAB Function2/1(d) -> d/1
  MATLAB Function2/2(angle) -> a/1
  MATLAB Function2/3(b) -> b/1, Scope/1

== system iq/best iq ==
  x : Inport  PortDimensions=4  SampleTime=1e-05
      mask Display: e = 0.06;c1 = [120 230 180]/255;c2 = ([120 230 180]+0)/(256+128);c3 = ([120 230 180]+128)/(256+128);patch([0 1 1 0],[0 0 1 1],c1);patch([0 1 1 1-e 1-e 0+e],[0 0 1 1-e 0+e 0+e],c2);patch([0 0 1 1-e 0+e 0+e],[0 1 1 1-e 1-e 0+e],c3);plot([0 1 1 0 0],[0 0 1 1 0]);
  Layer 1 : Subsystem
      mask Display: e = 0.06;c1 = [120 150 230]/255;c2 = ([120 150 230]+0)/383;c3 = ([120 150 230]+128)/383;patch([0 1 1 0],[0 0 1 1],c1);patch([0 1 1 1-e 1-e 0+e],[0 0 1 1-e 0+e 0+e],c2);patch([0 0 1 1-e 0+e 0+e],[0 1 1 1-e 1-e 0+e],c3);plot([0 1 1 0 0],[0 0 1 1 0]);
  Layer 2 : Subsystem
      mask Display: e = 0.06;c1 = [120 150 230]/255;c2 = ([120 150 230]+0)/383;c3 = ([120 150 230]+128)/383;patch([0 1 1 0],[0 0 1 1],c1);patch([0 1 1 1-e 1-e 0+e],[0 0 1 1-e 0+e 0+e],c2);patch([0 0 1 1-e 0+e 0+e],[0 1 1 1-e 1-e 0+e],c3);plot([0 1 1 0 0],[0 0 1 1 0]);
  Process Input 1 : Subsystem
      mask Display: e = 0.06;c1 = [120 150 230]/255;c2 = ([120 150 230]+0)/383;c3 = ([120 150 230]+128)/383;patch([0 1 1 0],[0 0 1 1],c1);patch([0 1 1 1-e 1-e 0+e],[0 0 1 1-e 0+e 0+e],c2);patch([0 0 1 1-e 0+e 0+e],[0 1 1 1-e 1-e 0+e],c3);plot([0 1 1 0 0],[0 0 1 1 0]);
  Process Output 1 : Subsystem
      mask Display: e = 0.06;c1 = [120 150 230]/255;c2 = ([120 150 230]+0)/383;c3 = ([120 150 230]+128)/383;patch([0 1 1 0],[0 0 1 1],c1);patch([0 1 1 1-e 1-e 0+e],[0 0 1 1-e 0+e 0+e],c2);patch([0 0 1 1-e 0+e 0+e],[0 1 1 1-e 1-e 0+e],c3);plot([0 1 1 0 0],[0 0 1 1 0]);
  y : Outport  InitialOutput=0
      mask Display: e = 0.06;c1 = [120 230 180]/255;c2 = ([120 230 180]+0)/(256+128);c3 = ([120 230 180]+128)/(256+128);patch([0 1 1 0],[0 0 1 1],c1);patch([0 1 1 1-e 1-e 0+e],[0 0 1 1-e 0+e 0+e],c2);patch([0 0 1 1-e 0+e 0+e],[0 1 1 1-e 1-e 0+e],c3);plot([0 1 1 0 0],[0 0 1 1 0]);
  wires:
  x/1 -> Process Input 1/1(x)
  Process Output 1/1(y) -> y/1
  Process Input 1/1(p) -> Layer 1/1("p{1}")
  Layer 1/1("a{1}") -> [feedback1]
  [feedback1] -> Layer 2/1("a{1} ")
  Layer 2/1("a{2}") -> [feedback2], Process Output 1/1(a)
  [feedback2] -> Layer 1/2("a{2} ")

== system iq/NARX Neural Network - Closed Loop/Layer 1 ==
  "p{1}" : Inport  PortDimensions=4  SampleTime=1e-05
      mask Display: e = 0.06;c1 = [120 230 180]/255;c2 = ([120 230 180]+0)/(256+128);c3 = ([120 230 180]+128)/(256+128);patch([0 1 1 0],[0 0 1 1],c1);patch([0 1 1 1-e 1-e 0+e],[0 0 1 1-e 0+e 0+e],c2);patch([0 0 1 1-e 0+e 0+e],[0 1 1 1-e 1-e 0+e],c3);plot([0 1 1 0 0],[0 0 1 1 0]);
  "a{2} " : Inport  Port=2  PortDimensions=1  SampleTime=1e-05
      mask Display: e = 0.06;c1 = [120 230 180]/255;c2 = ([120 230 180]+0)/(256+128);c3 = ([120 230 180]+128)/(256+128);patch([0 1 1 0],[0 0 1 1],c1);patch([0 1 1 1-e 1-e 0+e],[0 0 1 1-e 0+e 0+e],c2);patch([0 0 1 1-e 0+e 0+e],[0 1 1 1-e 1-e 0+e],c3);plot([0 1 1 0 0],[0 0 1 1 0]);
  Delays 1 : Subsystem
      mask Display: e = 0.06;c1 = [120 150 230]/255;c2 = ([120 150 230]+0)/383;c3 = ([120 150 230]+128)/383;patch([0 1 1 0],[0 0 1 1],c1);patch([0 1 1 1-e 1-e 0+e],[0 0 1 1-e 0+e 0+e],c2);patch([0 0 1 1-e 0+e 0+e],[0 1 1 1-e 1-e 0+e],c3);plot([0 1 1 0 0],[0 0 1 1 0]);disp('1-10');
  Delays 2 : Subsystem
      mask Display: e = 0.06;c1 = [120 150 230]/255;c2 = ([120 150 230]+0)/383;c3 = ([120 150 230]+128)/383;patch([0 1 1 0],[0 0 1 1],c1);patch([0 1 1 1-e 1-e 0+e],[0 0 1 1-e 0+e 0+e],c2);patch([0 0 1 1-e 0+e 0+e],[0 1 1 1-e 1-e 0+e],c3);plot([0 1 1 0 0],[0 0 1 1 0]);disp('1-10');
  "IW{1,1}" : Subsystem
      mask Display: e = 0.06;c1 = [120 150 230]/255;c2 = ([120 150 230]+0)/383;c3 = ([120 150 230]+128)/383;patch([0 1 1 0],[0 0 1 1],c1);patch([0 1 1 1-e 1-e 0+e],[0 0 1 1-e 0+e 0+e],c2);patch([0 0 1 1-e 0+e 0+e],[0 1 1 1-e 1-e 0+e],c3);plot([0 1 1 0 0],[0 0 1 1 0]);disp('W');
  "LW{1,2}" : Subsystem
      mask Display: e = 0.06;c1 = [120 150 230]/255;c2 = ([120 150 230]+0)/383;c3 = ([120 150 230]+128)/383;patch([0 1 1 0],[0 0 1 1],c1);patch([0 1 1 1-e 1-e 0+e],[0 0 1 1-e 0+e 0+e],c2);patch([0 0 1 1-e 0+e 0+e],[0 1 1 1-e 1-e 0+e],c3);plot([0 1 1 0 0],[0 0 1 1 0]);disp('W');
  "b{1}" : Constant  Value=[-0.190302503342581530443311521594296209514141082763671875;0.349524450488268800807389879992115311324596405029296875;0.1918290331474762633323649652083986438810825347900390625;1.0916224676680961191976848567719571292400360107421875;-0.1560575252297913551036145918260444886982440948486328125;-0.67918768290542519405761368034291081130504608154296875;0.69703375070224626863790717834490351378917694091796875;0.1869085129811998979842968537923297844827175140380859375;-0.637610909108960566271662173676304519176483154296875;-0.1539834683410511162460210243807523511350154876708984375]
      mask Display: e = 0.06;c1 = [120 150 230]/255;c2 = ([120 150 230]+0)/383;c3 = ([120 150 230]+128)/383;patch([0 1 1 0],[0 0 1 1],c1);patch([0 1 1 1-e 1-e 0+e],[0 0 1 1-e 0+e 0+e],c2);patch([0 0 1 1-e 0+e 0+e],[0 1 1 1-e 1-e 0+e],c3);plot([0 1 1 0 0],[0 0 1 1 0]);disp('b');
  netsum : Sum  Inputs=3  InputSameDT=on  SaturateOnIntegerOverflow=on  OutDataTypeStr=Inherit: Same as first input
      mask Display: e = 0.06;c1 = [120 150 230]/255;c2 = ([120 150 230]+0)/383;c3 = ([120 150 230]+128)/383;patch([0 1 1 0],[0 0 1 1],c1);patch([0 1 1 1-e 1-e 0+e],[0 0 1 1-e 0+e 0+e],c2);patch([0 0 1 1-e 0+e 0+e],[0 1 1 1-e 1-e 0+e],c3);plot([0 1 1 0 0],[0 0 1 1 0]);disp('+');
  tansig : neural/Transfer Functions/tansig
  "a{1}" : Outport  InitialOutput=[0;0;0;0;0;0;0;0;0;0]
      mask Display: e = 0.06;c1 = [120 230 180]/255;c2 = ([120 230 180]+0)/(256+128);c3 = ([120 230 180]+128)/(256+128);patch([0 1 1 0],[0 0 1 1],c1);patch([0 1 1 1-e 1-e 0+e],[0 0 1 1-e 0+e 0+e],c2);patch([0 0 1 1-e 0+e 0+e],[0 1 1 1-e 1-e 0+e],c3);plot([0 1 1 0 0],[0 0 1 1 0]);
  wires:
  "p{1}"/1 -> Delays 1/1("p{1}")
  Delays 1/1("pd{1,1}") -> "IW{1,1}"/1("pd{1,1}")
  "IW{1,1}"/1("iz{1,1}") -> netsum/1
  "a{2} "/1 -> Delays 2/1("p{1}")
  Delays 2/1("pd{1,2}") -> "LW{1,2}"/1("ad{1,2}")
  "LW{1,2}"/1("lz{1,2}") -> netsum/2
  "b{1}"/1 -> netsum/3
  netsum/1 -> tansig/1
  tansig/1 -> "a{1}"/1

== system iq/NARX Neural Network - Closed Loop/Layer 2 ==
  "a{1} " : Inport  PortDimensions=10  SampleTime=1e-05
      mask Display: e = 0.06;c1 = [120 230 180]/255;c2 = ([120 230 180]+0)/(256+128);c3 = ([120 230 180]+128)/(256+128);patch([0 1 1 0],[0 0 1 1],c1);patch([0 1 1 1-e 1-e 0+e],[0 0 1 1-e 0+e 0+e],c2);patch([0 0 1 1-e 0+e 0+e],[0 1 1 1-e 1-e 0+e],c3);plot([0 1 1 0 0],[0 0 1 1 0]);
  Delays 1 : Subsystem
      mask Display: e = 0.06;c1 = [120 150 230]/255;c2 = ([120 150 230]+0)/383;c3 = ([120 150 230]+128)/383;patch([0 1 1 0],[0 0 1 1],c1);patch([0 1 1 1-e 1-e 0+e],[0 0 1 1-e 0+e 0+e],c2);patch([0 0 1 1-e 0+e 0+e],[0 1 1 1-e 1-e 0+e],c3);plot([0 1 1 0 0],[0 0 1 1 0]);disp('0');
  "LW{2,1}" : Subsystem
      mask Display: e = 0.06;c1 = [120 150 230]/255;c2 = ([120 150 230]+0)/383;c3 = ([120 150 230]+128)/383;patch([0 1 1 0],[0 0 1 1],c1);patch([0 1 1 1-e 1-e 0+e],[0 0 1 1-e 0+e 0+e],c2);patch([0 0 1 1-e 0+e 0+e],[0 1 1 1-e 1-e 0+e],c3);plot([0 1 1 0 0],[0 0 1 1 0]);disp('W');
  "b{2}" : Constant  Value=1.4780142198057875102534808320342563092708587646484375
      mask Display: e = 0.06;c1 = [120 150 230]/255;c2 = ([120 150 230]+0)/383;c3 = ([120 150 230]+128)/383;patch([0 1 1 0],[0 0 1 1],c1);patch([0 1 1 1-e 1-e 0+e],[0 0 1 1-e 0+e 0+e],c2);patch([0 0 1 1-e 0+e 0+e],[0 1 1 1-e 1-e 0+e],c3);plot([0 1 1 0 0],[0 0 1 1 0]);disp('b');
  netsum : Sum  Inputs=2  InputSameDT=on  SaturateOnIntegerOverflow=on  OutDataTypeStr=Inherit: Same as first input
      mask Display: e = 0.06;c1 = [120 150 230]/255;c2 = ([120 150 230]+0)/383;c3 = ([120 150 230]+128)/383;patch([0 1 1 0],[0 0 1 1],c1);patch([0 1 1 1-e 1-e 0+e],[0 0 1 1-e 0+e 0+e],c2);patch([0 0 1 1-e 0+e 0+e],[0 1 1 1-e 1-e 0+e],c3);plot([0 1 1 0 0],[0 0 1 1 0]);disp('+');
  purelin : neural/Transfer Functions/purelin
  "a{2}" : Outport  InitialOutput=0
      mask Display: e = 0.06;c1 = [120 230 180]/255;c2 = ([120 230 180]+0)/(256+128);c3 = ([120 230 180]+128)/(256+128);patch([0 1 1 0],[0 0 1 1],c1);patch([0 1 1 1-e 1-e 0+e],[0 0 1 1-e 0+e 0+e],c2);patch([0 0 1 1-e 0+e 0+e],[0 1 1 1-e 1-e 0+e],c3);plot([0 1 1 0 0],[0 0 1 1 0]);
  wires:
  "a{1} "/1 -> Delays 1/1("p{2}")
  Delays 1/1("pd{2,1}") -> "LW{2,1}"/1("ad{2,1}")
  "LW{2,1}"/1("lz{2,1}") -> netsum/1
  "b{2}"/1 -> netsum/2
  netsum/1 -> purelin/1
  purelin/1 -> "a{2}"/1

== system iq/NARX Neural Network - Closed Loop/Process Input 1 ==
  x : Inport  PortDimensions=4  SampleTime=1e-05
      mask Display: e = 0.06;c1 = [120 230 180]/255;c2 = ([120 230 180]+0)/(256+128);c3 = ([120 230 180]+128)/(256+128);patch([0 1 1 0],[0 0 1 1],c1);patch([0 1 1 1-e 1-e 0+e],[0 0 1 1-e 0+e 0+e],c2);patch([0 0 1 1-e 0+e 0+e],[0 1 1 1-e 1-e 0+e],c3);plot([0 1 1 0 0],[0 0 1 1 0]);
  mapminmax : neural/Processing Functions/mapminmax  xmin=[-1.46404176681774722545981148869;-1.6104098565772866358258852415;-1.03126728063155437276066095365;-1.03899224914709331635265243676]  xmax=[1.45898042234988922771776742593;1.61571241335278692474730632966;1.04495252271198157956177965389;1.03404832736378149427025618934]  ymin=-1  ymax=1
  p : Outport  PortDimensions=4  SampleTime=1e-05
      mask Display: e = 0.06;c1 = [120 230 180]/255;c2 = ([120 230 180]+0)/(256+128);c3 = ([120 230 180]+128)/(256+128);patch([0 1 1 0],[0 0 1 1],c1);patch([0 1 1 1-e 1-e 0+e],[0 0 1 1-e 0+e 0+e],c2);patch([0 0 1 1-e 0+e 0+e],[0 1 1 1-e 1-e 0+e],c3);plot([0 1 1 0 0],[0 0 1 1 0]);
  wires:
  x/1 -> mapminmax/1
  mapminmax/1 -> p/1

== system iq/NARX Neural Network - Closed Loop/Process Output 1 ==
  a : Inport  PortDimensions=1  SampleTime=1e-05
      mask Display: e = 0.06;c1 = [120 230 180]/255;c2 = ([120 230 180]+0)/(256+128);c3 = ([120 230 180]+128)/(256+128);patch([0 1 1 0],[0 0 1 1],c1);patch([0 1 1 1-e 1-e 0+e],[0 0 1 1-e 0+e 0+e],c2);patch([0 0 1 1-e 0+e 0+e],[0 1 1 1-e 1-e 0+e],c3);plot([0 1 1 0 0],[0 0 1 1 0]);
  mapminmax_reverse : neural/Processing Functions/mapminmax_reverse  xmin=-1.20997753620370951388451885578  xmax=1.18040572127041376582212706126  ymin=-1  ymax=1
  y : Outport  PortDimensions=1  SampleTime=1e-05
      mask Display: e = 0.06;c1 = [120 230 180]/255;c2 = ([120 230 180]+0)/(256+128);c3 = ([120 230 180]+128)/(256+128);patch([0 1 1 0],[0 0 1 1],c1);patch([0 1 1 1-e 1-e 0+e],[0 0 1 1-e 0+e 0+e],c2);patch([0 0 1 1-e 0+e 0+e],[0 1 1 1-e 1-e 0+e],c3);plot([0 1 1 0 0],[0 0 1 1 0]);
  wires:
  a/1 -> mapminmax_reverse/1
  mapminmax_reverse/1 -> y/1

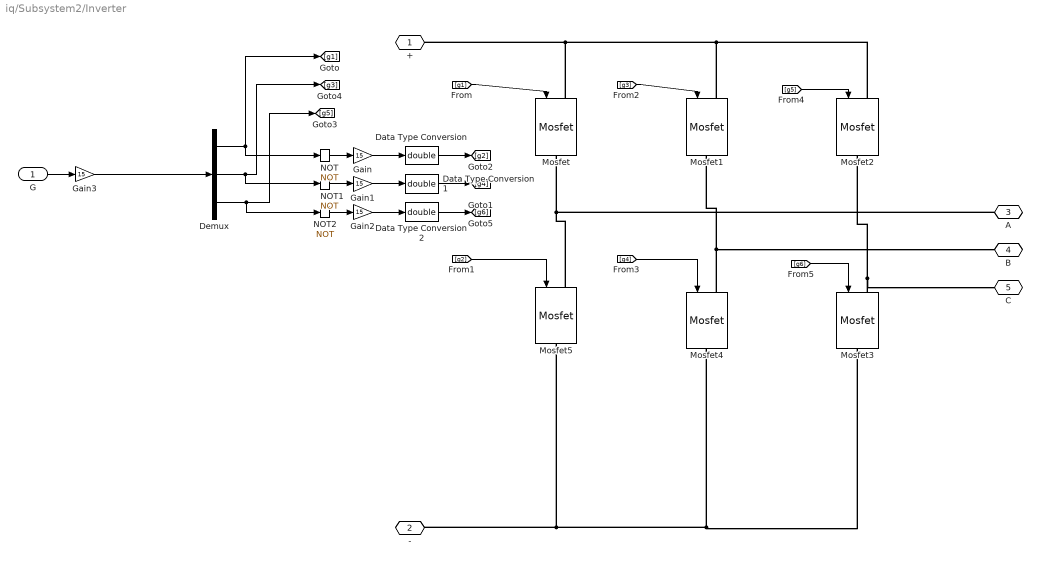
== system iq/Subsystem2/Inverter ==
  G : Inport
  Data Type Conversion : DataTypeConversion  OutDataTypeStr=double
  Data Type Conversion1 : DataTypeConversion  OutDataTypeStr=double
  Data Type Conversion2 : DataTypeConversion  OutDataTypeStr=double
  Demux : Demux  Outputs=3
  Gain{,1..3} (4 alike) : Gain  Gain=15
  Mosfet{,1..5} (6 alike) : spsMosfetLib/Mosfet  Ron=0.052  Lon=0  Rd=0.052  Vfd=0.8  IC=0  Rs=1e5  Cs=inf  Measurements=off
  NOT : Logic  Operator=NOT  IconShape=distinctive  AllPortsSameDT=off  OutDataTypeStr=boolean
  NOT1 : Logic  Operator=NOT  IconShape=distinctive  AllPortsSameDT=off  OutDataTypeStr=boolean
  NOT2 : Logic  Operator=NOT  IconShape=distinctive  AllPortsSameDT=off  OutDataTypeStr=boolean
  + : PMIOPort  Side=Left
  - : PMIOPort  Port=2  Side=Left
  A : PMIOPort  Port=3  Side=Right
  B : PMIOPort  Port=4  Side=Right
  C : PMIOPort  Port=5  Side=Right
  wires:
  [g2] -> Mosfet5/1
  [g6] -> Mosfet3/1
  [g1] -> Mosfet/1
  G/1 -> Gain3/1
  [g3] -> Mosfet1/1
  [g4] -> Mosfet4/1
  Demux/2 -> NOT1/1, [g3]
  Demux/3 -> NOT2/1, [g5]
  NOT/1 -> Gain/1
  NOT1/1 -> Gain1/1
  NOT2/1 -> Gain2/1
  Gain/1 -> Data Type Conversion/1
  Gain1/1 -> Data Type Conversion1/1
  Gain2/1 -> Data Type Conversion2/1
  Data Type Conversion/1 -> [g2]
  Data Type Conversion1/1 -> [g4]
  Data Type Conversion2/1 -> [g6]
  [g5] -> Mosfet2/1
  Gain3/1 -> Demux/1
  Demux/1 -> [g1], NOT/1
  connections:
  Mosfet/RConn1 -- Mosfet5/LConn1 -- A/RConn1
  Mosfet1/RConn1 -- B/RConn1 -- Mosfet4/LConn1
  Mosfet2/RConn1 -- C/RConn1 -- Mosfet3/LConn1
  Mosfet1/LConn1 -- Mosfet2/LConn1 -- Mosfet/LConn1 -- +/RConn1
  -/RConn1 -- Mosfet5/RConn1 -- Mosfet3/RConn1 -- Mosfet4/RConn1

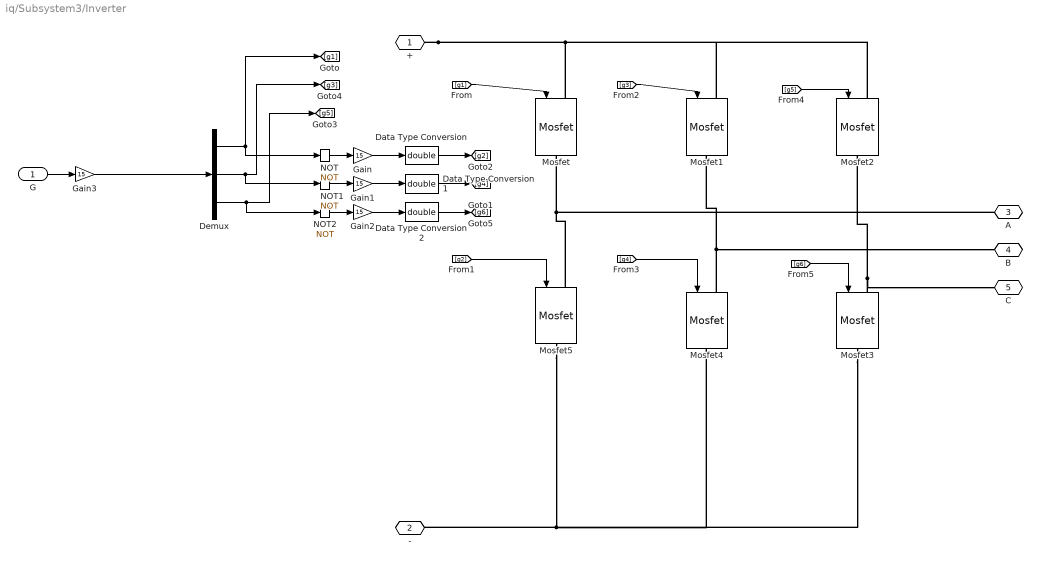
== system iq/Subsystem3/Inverter ==
  G : Inport
  Data Type Conversion : DataTypeConversion  OutDataTypeStr=double
  Data Type Conversion1 : DataTypeConversion  OutDataTypeStr=double
  Data Type Conversion2 : DataTypeConversion  OutDataTypeStr=double
  Demux : Demux  Outputs=3
  Gain{,1..3} (4 alike) : Gain  Gain=15
  Mosfet{,1..5} (6 alike) : spsMosfetLib/Mosfet  Ron=0.052  Lon=0  Rd=0.052  Vfd=0.8  IC=0  Rs=1e5  Cs=inf  Measurements=off
  NOT : Logic  Operator=NOT  IconShape=distinctive  AllPortsSameDT=off  OutDataTypeStr=boolean
  NOT1 : Logic  Operator=NOT  IconShape=distinctive  AllPortsSameDT=off  OutDataTypeStr=boolean
  NOT2 : Logic  Operator=NOT  IconShape=distinctive  AllPortsSameDT=off  OutDataTypeStr=boolean
  + : PMIOPort  Side=Left
  - : PMIOPort  Port=2  Side=Left
  A : PMIOPort  Port=3  Side=Right
  B : PMIOPort  Port=4  Side=Right
  C : PMIOPort  Port=5  Side=Right
  wires:
  Demux/1 -> NOT/1, [g1]
  Gain3/1 -> Demux/1
  [g5] -> Mosfet2/1
  Data Type Conversion2/1 -> [g6]
  Data Type Conversion1/1 -> [g4]
  Data Type Conversion/1 -> [g2]
  Gain2/1 -> Data Type Conversion2/1
  Gain1/1 -> Data Type Conversion1/1
  Gain/1 -> Data Type Conversion/1
  NOT2/1 -> Gain2/1
  NOT1/1 -> Gain1/1
  NOT/1 -> Gain/1
  Demux/3 -> [g5], NOT2/1
  Demux/2 -> [g3], NOT1/1
  [g4] -> Mosfet4/1
  [g3] -> Mosfet1/1
  G/1 -> Gain3/1
  [g1] -> Mosfet/1
  [g6] -> Mosfet3/1
  [g2] -> Mosfet5/1
  connections:
  Mosfet3/RConn1 -- Mosfet4/RConn1 -- Mosfet5/RConn1 -- -/RConn1
  +/RConn1 -- Mosfet/LConn1 -- Mosfet2/LConn1 -- Mosfet1/LConn1
  Mosfet3/LConn1 -- C/RConn1 -- Mosfet2/RConn1
  Mosfet4/LConn1 -- B/RConn1 -- Mosfet1/RConn1
  A/RConn1 -- Mosfet5/LConn1 -- Mosfet/RConn1
